simulink model "PhaseShifter"  (R2022b)
settings: Solver=VariableStepAuto  StartTime=0.0  StopTime=10.0  RelTol=1e-3
settings Model: Creator=mliu  LastModifiedBy=mliu

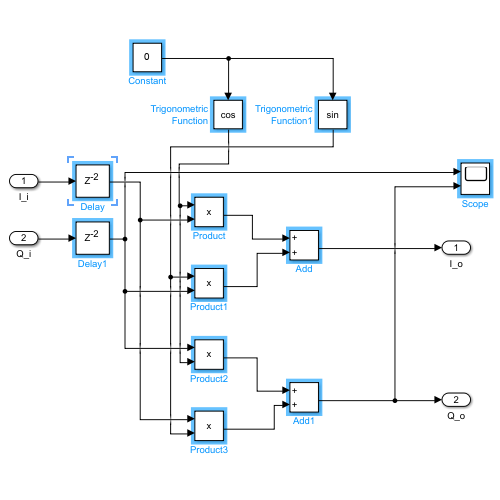
[thumbnail: Simulink's stored preview of the top-level diagram]
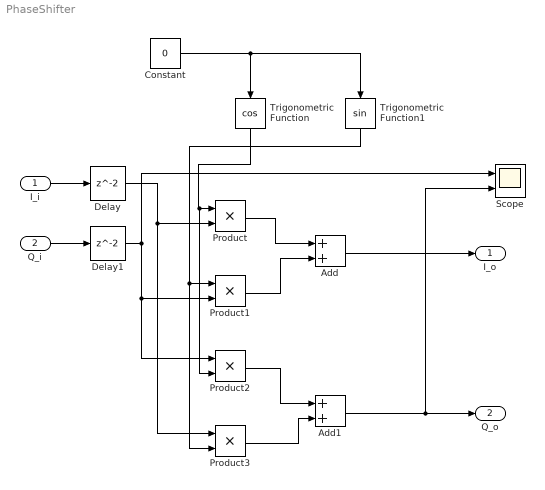
== system PhaseShifter ==
  I_i : Inport
  Q_i : Inport  Port=2
  Add : Sum
  Add1 : Sum
  Constant : Constant  Value=0
  Delay : Delay  InitialCondition=0
  Delay1 : Delay  InitialCondition=0
  Product{,1..3} (4 alike) : Product
  Scope : Scope  NumInputPorts=2
  Trigonometric Function : Trigonometry  Operator=cos
  Trigonometric Function1 : Trigonometry
  I_o : Outport
  Q_o : Outport  Port=2
  wires:
  I_i/1 -> Delay/1
  Q_i/1 -> Delay1/1
  Product/1 -> Add/1
  Product1/1 -> Add/2
  Product2/1 -> Add1/1
  Product3/1 -> Add1/2
  Add/1 -> I_o/1
  Add1/1 -> Scope/2, Q_o/1
  Constant/1 -> Trigonometric Function/1, Trigonometric Function1/1
  Trigonometric Function/1 -> Product2/2, Product/1
  Trigonometric Function1/1 -> Product3/2, Product1/1
  Delay/1 -> Product3/1, Product/2
  Delay1/1 -> Scope/1, Product2/1, Product1/2
